simulink model "takehome_111032552"  (R2022b)
settings: Solver=VariableStepAuto  StartTime=0.0  StopTime=20  RelTol=1e-3
libraries: slpidlib x4
settings Model: Creator=sheng  LastModifiedBy=sheng

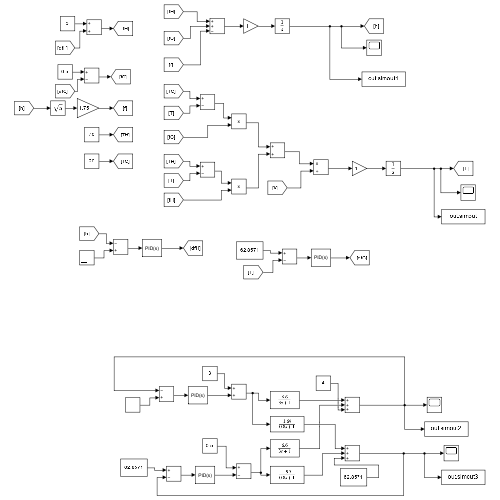
[thumbnail: Simulink's stored preview of the top-level diagram]
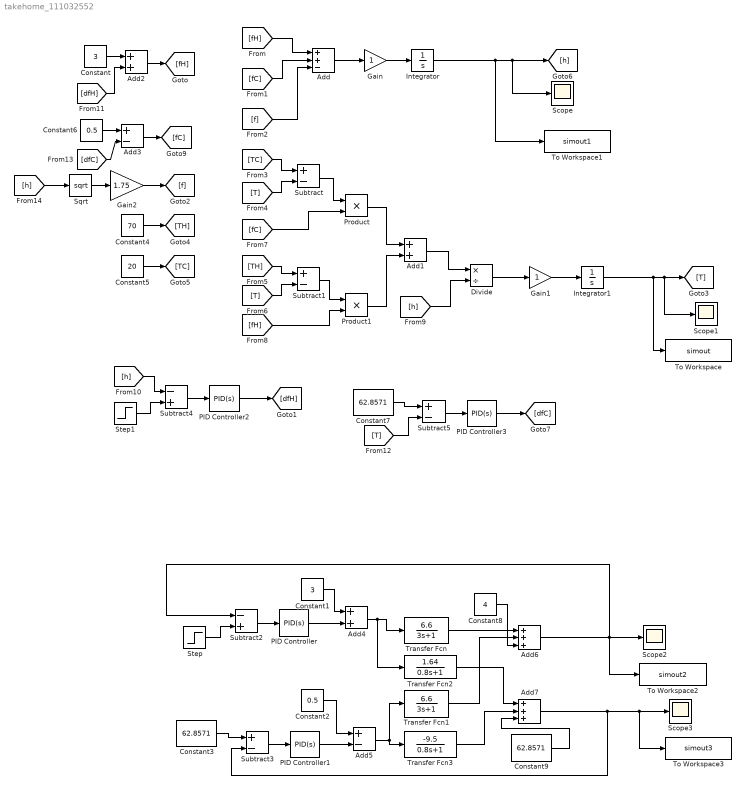
== system takehome_111032552 ==
  Add : Sum  Inputs=++-
  Add1 : Sum
  Add2 : Sum
  Add3 : Sum  Inputs=+-
  Add4 : Sum
  Add5 : Sum  Inputs=+-
  Add6 : Sum  Inputs=+++
  Add7 : Sum  Inputs=+++
  Constant : Constant  Value=3
  Constant1 : Constant  Value=3
  Constant2 : Constant  Value=0.5
  Constant3 : Constant  Value=62.8571
  Constant4 : Constant  Value=70
  Constant5 : Constant  Value=20
  Constant6 : Constant  Value=0.5
  Constant7 : Constant  Value=62.8571
  Constant8 : Constant  Value=4
  Constant9 : Constant  Value=62.8571
  Divide : Product  Inputs=*/
  Gain : Gain
  Gain1 : Gain
  Gain2 : Gain  Gain=1.75
  Integrator : Integrator  InitialCondition=4
  Integrator1 : Integrator  InitialCondition=62.8571
  PID Controller{,1..3} (4 alike) : slpidlib/PID Controller  Controller=PID  Form=Parallel  TimeDomain=Continuous-time  UseExternalTs=off  SampleTime=-1  IntegratorMethod=Forward Euler  FilterMethod=Forward Euler  ControllerParametersSource=internal  P=1  I=1  UseKiTs=off  D=0  N=100  UseFilter=on  TunerSelectOption=Transfer Function Based (PID Tuner App)  InitialConditionSource=internal  InitialConditionForIntegrator=0  InitialConditionForFilter=0  DifferentiatorICPrevScaledInput=0  ExternalReset=none  TrackingMode=off  Kt=1  LimitOutput=off  SatLimitsSource=internal  UpperSaturationLimit=inf  LowerSaturationLimit=-inf  LinearizeAsGain=on  AntiWindupMode=none  Kb=1  LimitIntegrator=off  UpperIntegratorSaturationLimit=inf  LowerIntegratorSaturationLimit=-inf  POutMin=[]  POutMax=[]  IOutMin=[]  IOutMax=[]  DOutMin=[]  DOutMax=[]  NOutMin=[]  NOutMax=[]  SumOutMin=[]  SumOutMax=[]  SaturationOutMin=[]  SaturationOutMax=[]  PParamMin=[]  PParamMax=[]  IParamMin=[]  IParamMax=[]  DParamMin=[]  DParamMax=[]  NParamMin=[]  NParamMax=[]  KbParamMin=[]  KbParamMax=[]  KtParamMin=[]  KtParamMax=[]  KbOutMin=[]  KbOutMax=[]  KtOutMin=[]  KtOutMax=[]  IntegratorOutMin=[]  IntegratorOutMax=[]  FilterOutMin=[]  FilterOutMax=[]  SumI1OutMin=[]  SumI1OutMax=[]  SumI2OutMin=[]  SumI2OutMax=[]  SumI3OutMin=[]  SumI3OutMax=[]  SumI4OutMin=[]  SumI4OutMax=[]  SumDOutMin=[]  SumDOutMax=[]  DifferentiatorOutMin=[]  DifferentiatorOutMax=[]  FilterDiffOutCoefMin=[]  FilterDiffOutCoefMax=[]  ReciprocalOutMin=[]  ReciprocalOutMax=[]  SumDenOutMin=[]  SumDenOutMax=[]  SumNumOutMin=[]  SumNumOutMax=[]  DivideOutMin=[]  DivideOutMax=[]  UdiffTsProdOutMin=[]  UdiffTsProdOutMax=[]  NTsProdOutMin=[]  NTsProdOutMax=[]  UintegralTsProdOutMin=[]  UintegralTsProdOutMax=[]  UngainTsProdOutMin=[]  UngainTsProdOutMax=[]  ClampingZeroOutDataTypeStr=Inherit: Inherit via back propagation  ClampingZeroOutMin=[]  ClampingZeroOutMax=[]  FilterDenConstantOutDataTypeStr=Inherit: Inherit via back propagation  FilterDenConstantOutMin=[]  FilterDenConstantOutMax=[]  PCopyOutDataTypeStr=Inherit: Inherit via back propagation  PCopyOutMin=[]  PCopyOutMax=[]  NCopyOutDataTypeStr=Inherit: Inherit via back propagation  NCopyOutMin=[]  NCopyOutMax=[]  IntegratorContinuousStateAttributes=''  IntegratorStateMustResolveToSignalObject=off  IntegratorRTWStateStorageClass=Auto  FilterContinuousStateAttributes=''  FilterStateMustResolveToSignalObject=off  FilterRTWStateStorageClass=Auto  ParallelPVariant=InternalParameters  IdealPVariant=Disabled  IVariant=InternalParameters  DVariant=InternalParameters  IntegratorVariant=Continuous  SatVariant=Disabled  AWVariant=Passthrough  PCopyVariant=Disabled  TRVariant=Disabled  FdbkBlocksVariant=Forward  IdealPFdbkVariant=Disabled  SatFdbkVariant=Disabled  DerivativeFilterVariant=ContFilter  NVariant=InternalParameters  NCopyVariant=Disabled  FilterICVariant=InternalICsFilter  IntegratorICVariant=InternalICs  ExternalResetVariant=Disabled  TRSumVariant=Passthrough  SumFdbkVariant=Disabled  SumVariant=Sum_PID  TsampFilterVariant=InternalTs  TsampNgainVariant=Passthrough  TsampIntegralVariant=Passthrough  ExternalSaturationOutDataTypeStr=Inherit: Same as second input
  Product : Product
  Product1 : Product
  Scope{,1..3} (4 alike) : Scope
  Sqrt : Sqrt
  Step : Step  Before=4  After=5  SampleTime=0
  Step1 : Step  Before=4  After=5  SampleTime=0
  Subtract{,1,3,5} (4 alike) : Sum  Inputs=+-
  Subtract2 : Sum  Inputs=-+
  Subtract4 : Sum  Inputs=-+
  To Workspace : ToWorkspace  VariableName=simout  SaveFormat=Timeseries  SampleTime=-1
  To Workspace1 : ToWorkspace  VariableName=simout1  SaveFormat=Timeseries  SampleTime=-1
  To Workspace2 : ToWorkspace  VariableName=simout2  SaveFormat=Timeseries  SampleTime=-1
  To Workspace3 : ToWorkspace  VariableName=simout3  SaveFormat=Timeseries  SampleTime=-1
  Transfer Fcn : TransferFcn  Numerator=[6.6]  Denominator=[3 1]
  Transfer Fcn1 : TransferFcn  Numerator=[6.6]  Denominator=[3 1]
  Transfer Fcn2 : TransferFcn  Numerator=[1.64]  Denominator=[0.8 1]
  Transfer Fcn3 : TransferFcn  Numerator=[-9.5]  Denominator=[0.8 1]
  wires:
  Constant4/1 -> [TH]
  Constant5/1 -> [TC]
  [fH] -> Add/1
  [fC] -> Add/2
  [f] -> Add/3
  Add/1 -> Gain/1
  Gain/1 -> Integrator/1
  Gain2/1 -> [f]
  [TC] -> Subtract/1
  [T] -> Subtract/2
  [TH] -> Subtract1/1
  [T] -> Subtract1/2
  Subtract/1 -> Product/1
  [fC] -> Product/2
  Subtract1/1 -> Product1/1
  [fH] -> Product1/2
  Product/1 -> Add1/1
  Product1/1 -> Add1/2
  Gain1/1 -> Integrator1/1
  Add1/1 -> Divide/1
  [h] -> Divide/2
  Divide/1 -> Gain1/1
  Subtract2/1 -> PID Controller/1
  PID Controller/1 -> Add4/2
  Add2/1 -> [fH]
  Constant/1 -> Add2/1
  Subtract3/1 -> PID Controller1/1
  Constant3/1 -> Subtract3/1
  Constant6/1 -> Add3/1
  Add3/1 -> [fC]
  PID Controller1/1 -> Add5/2
  [h] -> Sqrt/1
  Sqrt/1 -> Gain2/1
  Constant1/1 -> Add4/1
  Add4/1 -> Transfer Fcn2/1, Transfer Fcn/1
  Constant2/1 -> Add5/1
  Add5/1 -> Transfer Fcn1/1, Transfer Fcn3/1
  Transfer Fcn/1 -> Add6/1
  Transfer Fcn1/1 -> Add6/2
  Transfer Fcn2/1 -> Add7/1
  Transfer Fcn3/1 -> Add7/2
  Step/1 -> Subtract2/2
  Add7/1 -> Subtract3/2, To Workspace3/1, Scope3/1
  [dfH] -> Add2/2
  [dfC] -> Add3/2
  Subtract4/1 -> PID Controller2/1
  PID Controller2/1 -> [dfH]
  Step1/1 -> Subtract4/2
  [h] -> Subtract4/1
  Subtract5/1 -> PID Controller3/1
  Constant7/1 -> Subtract5/1
  PID Controller3/1 -> [dfC]
  [T] -> Subtract5/2
  Integrator/1 -> To Workspace1/1, Scope/1, [h]
  Integrator1/1 -> To Workspace/1, Scope1/1, [T]
  Constant8/1 -> Add6/3
  Constant9/1 -> Add7/3
  Add6/1 -> Subtract2/1, To Workspace2/1, Scope2/1
